simulink model "AUV"  (R2015a)
settings: Solver=ode1  StartTime=0.0  StopTime=20.0  FixedStep=0.1  RelTol=1e-3
libraries: simulink x1
settings Model: Creator=Martin  LastModifiedBy=Martin

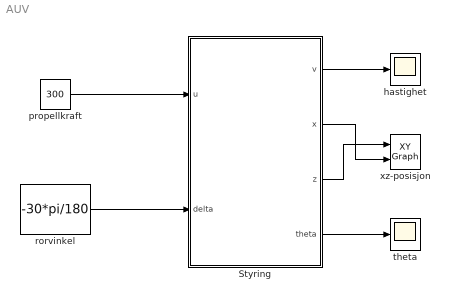
== system AUV ==
  Styring : Subsystem
  hastighet : Scope
  propellkraft : Constant  Value=300
  rorvinkel : Constant  Value=-30*pi/180
  theta : Scope
  xz-posisjon : simulink/Sinks/XY Graph  xmin=-100  xmax=100  ymin=-100  ymax=100  st=-1
  wires:
  propellkraft/1 -> Styring/1(u)
  rorvinkel/1 -> Styring/2(delta)
  Styring/1(v) -> hastighet/1
  Styring/2(x) -> xz-posisjon/2
  Styring/3(z) -> xz-posisjon/1
  Styring/4(theta) -> theta/1

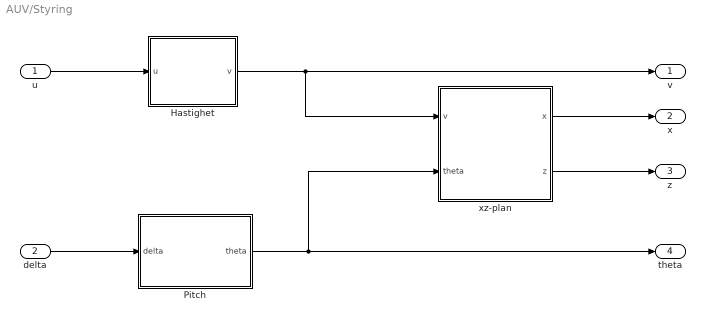
== system AUV/Styring ==
  u : Inport
  delta : Inport  Port=2
  Hastighet : Subsystem
  Pitch : Subsystem
  xz-plan : Subsystem
  v : Outport
  x : Outport  Port=2
  z : Outport  Port=3
  theta : Outport  Port=4
  wires:
  delta/1 -> Pitch/1(delta)
  xz-plan/2(z) -> z/1
  xz-plan/1(x) -> x/1
  Hastighet/1(v) -> v/1, xz-plan/1(v)
  Pitch/1(theta) -> theta/1, xz-plan/2(theta)
  u/1 -> Hastighet/1(u)

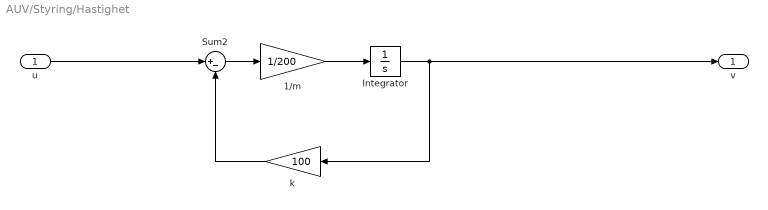
== system AUV/Styring/Hastighet ==
  u : Inport
  1/m : Gain  Gain=1/200
  "Integrator " : Integrator
  Sum2 : Sum  Inputs=|+-
  k : Gain  Gain=100
  v : Outport
  wires:
  Sum2/1 -> 1/m/1
  k/1 -> Sum2/2
  1/m/1 -> "Integrator "/1
  u/1 -> Sum2/1
  "Integrator "/1 -> v/1, k/1

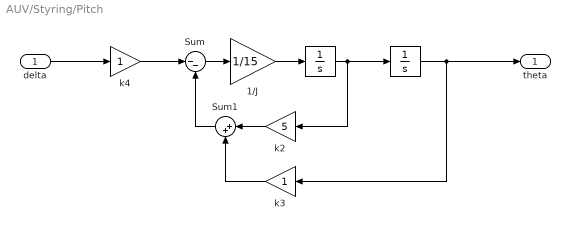
== system AUV/Styring/Pitch ==
  delta : Inport
  " " : Integrator
  "  " : Integrator
  1/J : Gain  Gain=1/15
  Sum : Sum  Inputs=|--
  Sum1 : Sum  Inputs=|++
  k2 : Gain  Gain=5
  k3 : Gain
  k4 : Gain
  theta : Outport
  wires:
  k2/1 -> Sum1/1
  delta/1 -> k4/1
  " "/1 -> k2/1, "  "/1
  Sum/1 -> 1/J/1
  k4/1 -> Sum/1
  1/J/1 -> " "/1
  k3/1 -> Sum1/2
  Sum1/1 -> Sum/2
  "  "/1 -> theta/1, k3/1

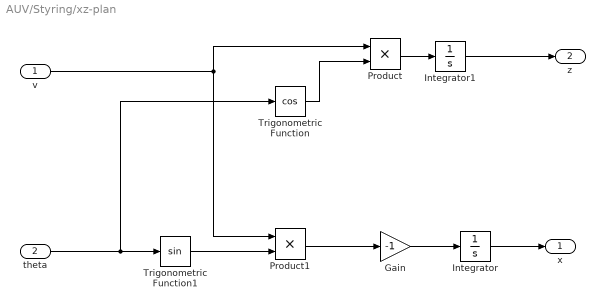
== system AUV/Styring/xz-plan ==
  v : Inport
  theta : Inport  Port=2
  Gain : Gain  Gain=-1
  Integrator : Integrator
  Integrator1 : Integrator
  Product : Product
  Product1 : Product
  Trigonometric Function : Trigonometry  Operator=cos
  Trigonometric Function1 : Trigonometry
  x : Outport
  z : Outport  Port=2
  wires:
  Integrator/1 -> x/1
  Trigonometric Function/1 -> Product/2
  Trigonometric Function1/1 -> Product1/2
  Product1/1 -> Gain/1
  v/1 -> Product1/1, Product/1
  Integrator1/1 -> z/1
  theta/1 -> Trigonometric Function/1, Trigonometric Function1/1
  Gain/1 -> Integrator/1
  Product/1 -> Integrator1/1
